simulink model "Lab1A_Task_4"  (R2019b)
settings: Solver=VariableStepAuto  StartTime=0.0  StopTime=60.0  RelTol=1e-3
settings Model: Creator=sinow  LastModifiedBy=sinow

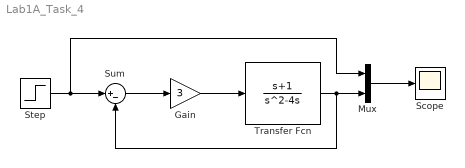
== system Lab1A_Task_4 ==
  Gain : Gain  Gain=3
  Mux : Mux  Inputs=2
  Scope : Scope
  Step : Step  Time=0  SampleTime=0
  Sum : Sum  Inputs=|+-
  Transfer Fcn : TransferFcn  Numerator=[1 1]  Denominator=[1 -4 0]
  wires:
  Step/1 -> Mux/1, Sum/1
  Sum/1 -> Gain/1
  Gain/1 -> Transfer Fcn/1
  Transfer Fcn/1 -> Mux/2, Sum/2
  Mux/1 -> Scope/1
